simulink model "controller_dev_sg_HIL_noTP"  (R2018b)
settings: configuration reference "Physics" (kept outside this file)
model workspace (MAT data in the model file):
  m = 1000
values from neighbouring files (symbols this model uses):
  bool_activate_Vehicles : value not decoded    [controller_dev_sg.sldd]
  ModObj_ObjList_SendPort = 11004.0    [UDPPortConfig.sldd]
  ModSens_GpsSenDat_SendPort = 3002.0    [UDPPortConfig.sldd]
  sensors_freq_camera = 37.0    [controller_dev_sg.sldd]
  sensors_freq_gps = 20.0    [controller_dev_sg.sldd]
  sensors_freq_imu = 100.0    [controller_dev_sg.sldd]
  sensors_freq_lidar = 12.0    [controller_dev_sg.sldd]
  sensors_freq_radar = 20.0    [controller_dev_sg.sldd]
undefined symbols (not defined in the file or in its folder): activate_VariableFriction, C, tpa_map_Reference, tSPhysics, x0_vehiclepos_start_veh1, x0_vehiclepos_start_veh10, x0_vehiclepos_start_veh2, x0_vehiclepos_start_veh3, x0_vehiclepos_start_veh4, x0_vehiclepos_start_veh5, x0_vehiclepos_start_veh6, x0_vehiclepos_start_veh7, x0_vehiclepos_start_veh8, x0_vehiclepos_start_veh9
libraries: xpcutilitieslib x273, xpcrtudplib x215, aerolibconvert2 x48, simulink x30, etargetslib x26, speedgoatlib_IO612 x7, canmsglib x6, slrtlib x4
(part 15 of 16)

== matlab function controller_dev_sg_HIL_noTP/UDP to Sensors (GNSS, IMU)/INSPVA/grid conv angle ==
  data: lat input; gamma output; lon input
function gamma = fcn(lat, lon)

gamma = grid_conv_angle(lat, lon);

== matlab function controller_dev_sg_HIL_noTP/UDP to Sensors (GNSS, IMU)1/INSPVA/CRC32 ==
  data: data input; crc output
function crc = fcn(data)

crc = crc32(data);

== matlab function controller_dev_sg_HIL_noTP/UDP to Sensors (GNSS, IMU)/INSPVA/normalizeAngle360 ==
  data: u input; y output
function y = fcn(u)

y = normalizeAngle360(u);

== matlab function controller_dev_sg_HIL_noTP/UDP to Sensors (GNSS, IMU)1/INSPVA/Header ==
  data: id input; first output; length input; time input; leapseconds input; second output; third output; hlength output; id output; type output; port output; mlength output; seq output; idletime output; timestatus output; week output; ms output; recstatus output; reserved output; version output
function [first, second, third, hlength, id, type, port, mlength, seq, idletime, timestatus, week, ms, recstatus, reserved, version] = fcn(id, length, time, leapseconds)

[first, second, third, hlength, id, type, port, mlength, seq, idletime, timestatus, week, ms, recstatus, reserved, version] = novatel_header(id, length, time, leapseconds);

== matlab function controller_dev_sg_HIL_noTP/UDP to Sensors (GNSS, IMU)1/INSPVA/grid conv angle ==
  data: lat input; gamma output; lon input
function gamma = fcn(lat, lon)

gamma = grid_conv_angle(lat, lon);

== matlab function controller_dev_sg_HIL_noTP/UDP to Sensors (GNSS, IMU)1/INSPVA/normalizeAngle360 ==
  data: u input; y output
function y = fcn(u)

y = normalizeAngle360(u);

== matlab function controller_dev_sg_HIL_noTP/UDP to Sensors (GNSS, IMU)1/INSPVA/tcs2llhT ==
  data: x input; lat output; y input; z input; origin input; lon output; hgt output
function [lat, lon, hgt]= fcn(x, y, z, origin)

llh =tcs2llhT([x; y; z], origin);
lat = llh(1,:);
lon = llh(2,:);
hgt = llh(3,:);
end

== matlab function controller_dev_sg_HIL_noTP/UDP to Sensors (GNSS, IMU)2/INSPVA/CRC32 ==
  data: data input; crc output
function crc = fcn(data)

crc = crc32(data);

== matlab function controller_dev_sg_HIL_noTP/UDP to Sensors (GNSS, IMU)2/INSPVA/Header ==
  data: id input; first output; length input; time input; leapseconds input; second output; third output; hlength output; id output; type output; port output; mlength output; seq output; idletime output; timestatus output; week output; ms output; recstatus output; reserved output; version output
function [first, second, third, hlength, id, type, port, mlength, seq, idletime, timestatus, week, ms, recstatus, reserved, version] = fcn(id, length, time, leapseconds)

[first, second, third, hlength, id, type, port, mlength, seq, idletime, timestatus, week, ms, recstatus, reserved, version] = novatel_header(id, length, time, leapseconds);

== matlab function controller_dev_sg_HIL_noTP/UDP to Sensors (GNSS, IMU)2/INSPVA/grid conv angle ==
  data: lat input; gamma output; lon input
function gamma = fcn(lat, lon)

gamma = grid_conv_angle(lat, lon);

== matlab function controller_dev_sg_HIL_noTP/UDP to Sensors (GNSS, IMU)2/INSPVA/normalizeAngle360 ==
  data: u input; y output
function y = fcn(u)

y = normalizeAngle360(u);

== matlab function controller_dev_sg_HIL_noTP/UDP to Sensors (GNSS, IMU)2/INSPVA/tcs2llhT ==
  data: x input; lat output; y input; z input; origin input; lon output; hgt output
function [lat, lon, hgt]= fcn(x, y, z, origin)

llh =tcs2llhT([x; y; z], origin);
lat = llh(1,:);
lon = llh(2,:);
hgt = llh(3,:);
end

== matlab function controller_dev_sg_HIL_noTP/UDP to Sensors (GNSS, IMU)3/INSPVA/CRC32 ==
  data: data input; crc output
function crc = fcn(data)

crc = crc32(data);

== matlab function controller_dev_sg_HIL_noTP/UDP to Sensors (GNSS, IMU)3/INSPVA/Header ==
  data: id input; first output; length input; time input; leapseconds input; second output; third output; hlength output; id output; type output; port output; mlength output; seq output; idletime output; timestatus output; week output; ms output; recstatus output; reserved output; version output
function [first, second, third, hlength, id, type, port, mlength, seq, idletime, timestatus, week, ms, recstatus, reserved, version] = fcn(id, length, time, leapseconds)

[first, second, third, hlength, id, type, port, mlength, seq, idletime, timestatus, week, ms, recstatus, reserved, version] = novatel_header(id, length, time, leapseconds);

== matlab function controller_dev_sg_HIL_noTP/UDP to Sensors (GNSS, IMU)3/INSPVA/grid conv angle ==
  data: lat input; gamma output; lon input
function gamma = fcn(lat, lon)

gamma = grid_conv_angle(lat, lon);

== matlab function controller_dev_sg_HIL_noTP/UDP to Sensors (GNSS, IMU)3/INSPVA/normalizeAngle360 ==
  data: u input; y output
function y = fcn(u)

y = normalizeAngle360(u);

== matlab function controller_dev_sg_HIL_noTP/UDP to Sensors (GNSS, IMU)3/INSPVA/tcs2llhT ==
  data: x input; lat output; y input; z input; origin input; lon output; hgt output
function [lat, lon, hgt]= fcn(x, y, z, origin)

llh =tcs2llhT([x; y; z], origin);
lat = llh(1,:);
lon = llh(2,:);
hgt = llh(3,:);
end

== matlab function controller_dev_sg_HIL_noTP/UDP to Sensors (GNSS, IMU)4/INSPVA/CRC32 ==
  data: data input; crc output
function crc = fcn(data)

crc = crc32(data);

== matlab function controller_dev_sg_HIL_noTP/UDP to Sensors (GNSS, IMU)4/INSPVA/Header ==
  data: id input; first output; length input; time input; leapseconds input; second output; third output; hlength output; id output; type output; port output; mlength output; seq output; idletime output; timestatus output; week output; ms output; recstatus output; reserved output; version output
function [first, second, third, hlength, id, type, port, mlength, seq, idletime, timestatus, week, ms, recstatus, reserved, version] = fcn(id, length, time, leapseconds)

[first, second, third, hlength, id, type, port, mlength, seq, idletime, timestatus, week, ms, recstatus, reserved, version] = novatel_header(id, length, time, leapseconds);

== matlab function controller_dev_sg_HIL_noTP/UDP to Sensors (GNSS, IMU)4/INSPVA/grid conv angle ==
  data: lat input; gamma output; lon input
function gamma = fcn(lat, lon)

gamma = grid_conv_angle(lat, lon);

== matlab function controller_dev_sg_HIL_noTP/UDP to Sensors (GNSS, IMU)4/INSPVA/normalizeAngle360 ==
  data: u input; y output
function y = fcn(u)

y = normalizeAngle360(u);

== matlab function controller_dev_sg_HIL_noTP/UDP to Sensors (GNSS, IMU)4/INSPVA/tcs2llhT ==
  data: x input; lat output; y input; z input; origin input; lon output; hgt output
function [lat, lon, hgt]= fcn(x, y, z, origin)

llh =tcs2llhT([x; y; z], origin);
lat = llh(1,:);
lon = llh(2,:);
hgt = llh(3,:);
end

== matlab function controller_dev_sg_HIL_noTP/UDP to Sensors (GNSS, IMU)5/INSPVA/CRC32 ==
  data: data input; crc output
function crc = fcn(data)

crc = crc32(data);

== matlab function controller_dev_sg_HIL_noTP/UDP to Sensors (GNSS, IMU)5/INSPVA/Header ==
  data: id input; first output; length input; time input; leapseconds input; second output; third output; hlength output; id output; type output; port output; mlength output; seq output; idletime output; timestatus output; week output; ms output; recstatus output; reserved output; version output
function [first, second, third, hlength, id, type, port, mlength, seq, idletime, timestatus, week, ms, recstatus, reserved, version] = fcn(id, length, time, leapseconds)

[first, second, third, hlength, id, type, port, mlength, seq, idletime, timestatus, week, ms, recstatus, reserved, version] = novatel_header(id, length, time, leapseconds);

== matlab function controller_dev_sg_HIL_noTP/UDP to Sensors (GNSS, IMU)5/INSPVA/grid conv angle ==
  data: lat input; gamma output; lon input
function gamma = fcn(lat, lon)

gamma = grid_conv_angle(lat, lon);

== matlab function controller_dev_sg_HIL_noTP/UDP to Sensors (GNSS, IMU)5/INSPVA/normalizeAngle360 ==
  data: u input; y output
function y = fcn(u)

y = normalizeAngle360(u);

== matlab function controller_dev_sg_HIL_noTP/UDP to Sensors (GNSS, IMU)5/INSPVA/tcs2llhT ==
  data: x input; lat output; y input; z input; origin input; lon output; hgt output
function [lat, lon, hgt]= fcn(x, y, z, origin)

llh =tcs2llhT([x; y; z], origin);
lat = llh(1,:);
lon = llh(2,:);
hgt = llh(3,:);
end

== matlab function controller_dev_sg_HIL_noTP/UDP to Sensors (GNSS, IMU)6/INSPVA/CRC32 ==
  data: data input; crc output
function crc = fcn(data)

crc = crc32(data);

== matlab function controller_dev_sg_HIL_noTP/UDP to Sensors (GNSS, IMU)6/INSPVA/Header ==
  data: id input; first output; length input; time input; leapseconds input; second output; third output; hlength output; id output; type output; port output; mlength output; seq output; idletime output; timestatus output; week output; ms output; recstatus output; reserved output; version output
function [first, second, third, hlength, id, type, port, mlength, seq, idletime, timestatus, week, ms, recstatus, reserved, version] = fcn(id, length, time, leapseconds)

[first, second, third, hlength, id, type, port, mlength, seq, idletime, timestatus, week, ms, recstatus, reserved, version] = novatel_header(id, length, time, leapseconds);

== matlab function controller_dev_sg_HIL_noTP/UDP to Sensors (GNSS, IMU)6/INSPVA/grid conv angle ==
  data: lat input; gamma output; lon input
function gamma = fcn(lat, lon)

gamma = grid_conv_angle(lat, lon);

== matlab function controller_dev_sg_HIL_noTP/UDP to Sensors (GNSS, IMU)6/INSPVA/normalizeAngle360 ==
  data: u input; y output
function y = fcn(u)

y = normalizeAngle360(u);

== matlab function controller_dev_sg_HIL_noTP/UDP to Sensors (GNSS, IMU)6/INSPVA/tcs2llhT ==
  data: x input; lat output; y input; z input; origin input; lon output; hgt output
function [lat, lon, hgt]= fcn(x, y, z, origin)

llh =tcs2llhT([x; y; z], origin);
lat = llh(1,:);
lon = llh(2,:);
hgt = llh(3,:);
end

== matlab function controller_dev_sg_HIL_noTP/UDP to Sensors (GNSS, IMU)7/INSPVA/CRC32 ==
  data: data input; crc output
function crc = fcn(data)

crc = crc32(data);

== matlab function controller_dev_sg_HIL_noTP/UDP to Sensors (GNSS, IMU)7/INSPVA/Header ==
  data: id input; first output; length input; time input; leapseconds input; second output; third output; hlength output; id output; type output; port output; mlength output; seq output; idletime output; timestatus output; week output; ms output; recstatus output; reserved output; version output
function [first, second, third, hlength, id, type, port, mlength, seq, idletime, timestatus, week, ms, recstatus, reserved, version] = fcn(id, length, time, leapseconds)

[first, second, third, hlength, id, type, port, mlength, seq, idletime, timestatus, week, ms, recstatus, reserved, version] = novatel_header(id, length, time, leapseconds);

== matlab function controller_dev_sg_HIL_noTP/UDP to Sensors (GNSS, IMU)7/INSPVA/grid conv angle ==
  data: lat input; gamma output; lon input
function gamma = fcn(lat, lon)

gamma = grid_conv_angle(lat, lon);

== matlab function controller_dev_sg_HIL_noTP/UDP to Sensors (GNSS, IMU)7/INSPVA/normalizeAngle360 ==
  data: u input; y output
function y = fcn(u)

y = normalizeAngle360(u);

== matlab function controller_dev_sg_HIL_noTP/UDP to Sensors (GNSS, IMU)7/INSPVA/tcs2llhT ==
  data: x input; lat output; y input; z input; origin input; lon output; hgt output
function [lat, lon, hgt]= fcn(x, y, z, origin)

llh =tcs2llhT([x; y; z], origin);
lat = llh(1,:);
lon = llh(2,:);
hgt = llh(3,:);
end

== matlab function controller_dev_sg_HIL_noTP/UDP to Sensors (GNSS, IMU)/RAWIMU/CRC32 ==
  data: data input; crc output
function crc = fcn(data)

crc = crc32(data);

== matlab function controller_dev_sg_HIL_noTP/UDP to Sensors (GNSS, IMU)1/RAWIMU/CRC32 ==
  data: data input; crc output
function crc = fcn(data)

crc = crc32(data);

== matlab function controller_dev_sg_HIL_noTP/UDP to Sensors (GNSS, IMU)2/RAWIMU/CRC32 ==
  data: data input; crc output
function crc = fcn(data)

crc = crc32(data);

== matlab function controller_dev_sg_HIL_noTP/UDP to Sensors (GNSS, IMU)3/RAWIMU/CRC32 ==
  data: data input; crc output
function crc = fcn(data)

crc = crc32(data);

== matlab function controller_dev_sg_HIL_noTP/UDP to Sensors (GNSS, IMU)4/RAWIMU/CRC32 ==
  data: data input; crc output
function crc = fcn(data)

crc = crc32(data);

== matlab function controller_dev_sg_HIL_noTP/UDP to Sensors (GNSS, IMU)5/RAWIMU/CRC32 ==
  data: data input; crc output
function crc = fcn(data)

crc = crc32(data);

== matlab function controller_dev_sg_HIL_noTP/UDP to Sensors (GNSS, IMU)6/RAWIMU/CRC32 ==
  data: data input; crc output
function crc = fcn(data)

crc = crc32(data);

== matlab function controller_dev_sg_HIL_noTP/UDP to Sensors (GNSS, IMU)7/RAWIMU/CRC32 ==
  data: data input; crc output
function crc = fcn(data)

crc = crc32(data);

== matlab function controller_dev_sg_HIL_noTP/UDP to Sensors (GNSS, IMU)/BESTPOS/CRC1 ==
  data: data input; crc output
function crc = fcn(data)

crc = crc32(data);

== matlab function controller_dev_sg_HIL_noTP/UDP to Sensors (GNSS, IMU)/BESTPOS/Header1 ==
  data: id input; first output; length input; time input; leapseconds input; second output; third output; hlength output; id output; type output; port output; mlength output; seq output; idletime output; timestatus output; week output; ms output; recstatus output; reserved output; version output
function [first, second, third, hlength, id, type, port, mlength, seq, idletime, timestatus, week, ms, recstatus, reserved, version] = fcn(id, length, time, leapseconds)

[first, second, third, hlength, id, type, port, mlength, seq, idletime, timestatus, week, ms, recstatus, reserved, version] = novatel_header(id, length, time, leapseconds);

== matlab function controller_dev_sg_HIL_noTP/UDP to Sensors (GNSS, IMU)/BESTPOS/tcs2llhT1 ==
  data: x input; lat output; y input; z input; origin input; lon output; hgt output
function [lat, lon, hgt]= fcn(x, y, z, origin)

llh =tcs2llhT([x; y; z], origin);
lat = llh(1,:);
lon = llh(2,:);
hgt = llh(3,:);
end

== matlab function controller_dev_sg_HIL_noTP/UDP to Sensors (GNSS, IMU)1/BESTPOS/Header1 ==
  data: id input; first output; length input; time input; leapseconds input; second output; third output; hlength output; id output; type output; port output; mlength output; seq output; idletime output; timestatus output; week output; ms output; recstatus output; reserved output; version output
function [first, second, third, hlength, id, type, port, mlength, seq, idletime, timestatus, week, ms, recstatus, reserved, version] = fcn(id, length, time, leapseconds)

[first, second, third, hlength, id, type, port, mlength, seq, idletime, timestatus, week, ms, recstatus, reserved, version] = novatel_header(id, length, time, leapseconds);

== matlab function controller_dev_sg_HIL_noTP/UDP to Sensors (GNSS, IMU)1/BESTPOS/tcs2llhT ==
  data: x input; lat output; y input; z input; origin input; lon output; hgt output
function [lat, lon, hgt]= fcn(x, y, z, origin)

llh =tcs2llhT([x; y; z], origin);
lat = llh(1,:);
lon = llh(2,:);
hgt = llh(3,:);
end

== matlab function controller_dev_sg_HIL_noTP/UDP to Sensors (GNSS, IMU)1/BESTPOS/tcs2llhT1 ==
  data: x input; lat output; y input; z input; origin input; lon output; hgt output
function [lat, lon, hgt]= fcn(x, y, z, origin)

llh =tcs2llhT([x; y; z], origin);
lat = llh(1,:);
lon = llh(2,:);
hgt = llh(3,:);
end

== matlab function controller_dev_sg_HIL_noTP/UDP to Sensors (GNSS, IMU)2/BESTPOS/Header1 ==
  data: id input; first output; length input; time input; leapseconds input; second output; third output; hlength output; id output; type output; port output; mlength output; seq output; idletime output; timestatus output; week output; ms output; recstatus output; reserved output; version output
function [first, second, third, hlength, id, type, port, mlength, seq, idletime, timestatus, week, ms, recstatus, reserved, version] = fcn(id, length, time, leapseconds)

[first, second, third, hlength, id, type, port, mlength, seq, idletime, timestatus, week, ms, recstatus, reserved, version] = novatel_header(id, length, time, leapseconds);

== matlab function controller_dev_sg_HIL_noTP/UDP to Sensors (GNSS, IMU)2/BESTPOS/tcs2llhT ==
  data: x input; lat output; y input; z input; origin input; lon output; hgt output
function [lat, lon, hgt]= fcn(x, y, z, origin)

llh =tcs2llhT([x; y; z], origin);
lat = llh(1,:);
lon = llh(2,:);
hgt = llh(3,:);
end

== matlab function controller_dev_sg_HIL_noTP/UDP to Sensors (GNSS, IMU)2/BESTPOS/tcs2llhT1 ==
  data: x input; lat output; y input; z input; origin input; lon output; hgt output
function [lat, lon, hgt]= fcn(x, y, z, origin)

llh =tcs2llhT([x; y; z], origin);
lat = llh(1,:);
lon = llh(2,:);
hgt = llh(3,:);
end

== matlab function controller_dev_sg_HIL_noTP/UDP to Sensors (GNSS, IMU)3/BESTPOS/Header1 ==
  data: id input; first output; length input; time input; leapseconds input; second output; third output; hlength output; id output; type output; port output; mlength output; seq output; idletime output; timestatus output; week output; ms output; recstatus output; reserved output; version output
function [first, second, third, hlength, id, type, port, mlength, seq, idletime, timestatus, week, ms, recstatus, reserved, version] = fcn(id, length, time, leapseconds)

[first, second, third, hlength, id, type, port, mlength, seq, idletime, timestatus, week, ms, recstatus, reserved, version] = novatel_header(id, length, time, leapseconds);

== matlab function controller_dev_sg_HIL_noTP/UDP to Sensors (GNSS, IMU)3/BESTPOS/tcs2llhT ==
  data: x input; lat output; y input; z input; origin input; lon output; hgt output
function [lat, lon, hgt]= fcn(x, y, z, origin)

llh =tcs2llhT([x; y; z], origin);
lat = llh(1,:);
lon = llh(2,:);
hgt = llh(3,:);
end

== matlab function controller_dev_sg_HIL_noTP/UDP to Sensors (GNSS, IMU)3/BESTPOS/tcs2llhT1 ==
  data: x input; lat output; y input; z input; origin input; lon output; hgt output
function [lat, lon, hgt]= fcn(x, y, z, origin)

llh =tcs2llhT([x; y; z], origin);
lat = llh(1,:);
lon = llh(2,:);
hgt = llh(3,:);
end

== matlab function controller_dev_sg_HIL_noTP/UDP to Sensors (GNSS, IMU)4/BESTPOS/Header1 ==
  data: id input; first output; length input; time input; leapseconds input; second output; third output; hlength output; id output; type output; port output; mlength output; seq output; idletime output; timestatus output; week output; ms output; recstatus output; reserved output; version output
function [first, second, third, hlength, id, type, port, mlength, seq, idletime, timestatus, week, ms, recstatus, reserved, version] = fcn(id, length, time, leapseconds)

[first, second, third, hlength, id, type, port, mlength, seq, idletime, timestatus, week, ms, recstatus, reserved, version] = novatel_header(id, length, time, leapseconds);

== matlab function controller_dev_sg_HIL_noTP/UDP to Sensors (GNSS, IMU)4/BESTPOS/tcs2llhT ==
  data: x input; lat output; y input; z input; origin input; lon output; hgt output
function [lat, lon, hgt]= fcn(x, y, z, origin)

llh =tcs2llhT([x; y; z], origin);
lat = llh(1,:);
lon = llh(2,:);
hgt = llh(3,:);
end

== matlab function controller_dev_sg_HIL_noTP/UDP to Sensors (GNSS, IMU)4/BESTPOS/tcs2llhT1 ==
  data: x input; lat output; y input; z input; origin input; lon output; hgt output
function [lat, lon, hgt]= fcn(x, y, z, origin)

llh =tcs2llhT([x; y; z], origin);
lat = llh(1,:);
lon = llh(2,:);
hgt = llh(3,:);
end

== matlab function controller_dev_sg_HIL_noTP/UDP to Sensors (GNSS, IMU)5/BESTPOS/Header1 ==
  data: id input; first output; length input; time input; leapseconds input; second output; third output; hlength output; id output; type output; port output; mlength output; seq output; idletime output; timestatus output; week output; ms output; recstatus output; reserved output; version output
function [first, second, third, hlength, id, type, port, mlength, seq, idletime, timestatus, week, ms, recstatus, reserved, version] = fcn(id, length, time, leapseconds)

[first, second, third, hlength, id, type, port, mlength, seq, idletime, timestatus, week, ms, recstatus, reserved, version] = novatel_header(id, length, time, leapseconds);

== matlab function controller_dev_sg_HIL_noTP/UDP to Sensors (GNSS, IMU)5/BESTPOS/tcs2llhT ==
  data: x input; lat output; y input; z input; origin input; lon output; hgt output
function [lat, lon, hgt]= fcn(x, y, z, origin)

llh =tcs2llhT([x; y; z], origin);
lat = llh(1,:);
lon = llh(2,:);
hgt = llh(3,:);
end

== matlab function controller_dev_sg_HIL_noTP/UDP to Sensors (GNSS, IMU)5/BESTPOS/tcs2llhT1 ==
  data: x input; lat output; y input; z input; origin input; lon output; hgt output
function [lat, lon, hgt]= fcn(x, y, z, origin)

llh =tcs2llhT([x; y; z], origin);
lat = llh(1,:);
lon = llh(2,:);
hgt = llh(3,:);
end

== matlab function controller_dev_sg_HIL_noTP/UDP to Sensors (GNSS, IMU)6/BESTPOS/Header1 ==
  data: id input; first output; length input; time input; leapseconds input; second output; third output; hlength output; id output; type output; port output; mlength output; seq output; idletime output; timestatus output; week output; ms output; recstatus output; reserved output; version output
function [first, second, third, hlength, id, type, port, mlength, seq, idletime, timestatus, week, ms, recstatus, reserved, version] = fcn(id, length, time, leapseconds)

[first, second, third, hlength, id, type, port, mlength, seq, idletime, timestatus, week, ms, recstatus, reserved, version] = novatel_header(id, length, time, leapseconds);

== matlab function controller_dev_sg_HIL_noTP/UDP to Sensors (GNSS, IMU)6/BESTPOS/tcs2llhT ==
  data: x input; lat output; y input; z input; origin input; lon output; hgt output
function [lat, lon, hgt]= fcn(x, y, z, origin)

llh =tcs2llhT([x; y; z], origin);
lat = llh(1,:);
lon = llh(2,:);
hgt = llh(3,:);
end

== matlab function controller_dev_sg_HIL_noTP/UDP to Sensors (GNSS, IMU)6/BESTPOS/tcs2llhT1 ==
  data: x input; lat output; y input; z input; origin input; lon output; hgt output
function [lat, lon, hgt]= fcn(x, y, z, origin)

llh =tcs2llhT([x; y; z], origin);
lat = llh(1,:);
lon = llh(2,:);
hgt = llh(3,:);
end

== matlab function controller_dev_sg_HIL_noTP/UDP to Sensors (GNSS, IMU)7/BESTPOS/Header1 ==
  data: id input; first output; length input; time input; leapseconds input; second output; third output; hlength output; id output; type output; port output; mlength output; seq output; idletime output; timestatus output; week output; ms output; recstatus output; reserved output; version output
function [first, second, third, hlength, id, type, port, mlength, seq, idletime, timestatus, week, ms, recstatus, reserved, version] = fcn(id, length, time, leapseconds)

[first, second, third, hlength, id, type, port, mlength, seq, idletime, timestatus, week, ms, recstatus, reserved, version] = novatel_header(id, length, time, leapseconds);

== matlab function controller_dev_sg_HIL_noTP/UDP to Sensors (GNSS, IMU)7/BESTPOS/tcs2llhT ==
  data: x input; lat output; y input; z input; origin input; lon output; hgt output
function [lat, lon, hgt]= fcn(x, y, z, origin)

llh =tcs2llhT([x; y; z], origin);
lat = llh(1,:);
lon = llh(2,:);
hgt = llh(3,:);
end

== matlab function controller_dev_sg_HIL_noTP/UDP to Sensors (GNSS, IMU)7/BESTPOS/tcs2llhT1 ==
  data: x input; lat output; y input; z input; origin input; lon output; hgt output
function [lat, lon, hgt]= fcn(x, y, z, origin)

llh =tcs2llhT([x; y; z], origin);
lat = llh(1,:);
lon = llh(2,:);
hgt = llh(3,:);
end

== matlab function controller_dev_sg_HIL_noTP/UDP to Sensors (GNSS, IMU)/DUALANTENNAHEADING/CRC32 ==
  data: data input; crc output
function crc = fcn(data)

crc = crc32(data);

== matlab function controller_dev_sg_HIL_noTP/UDP to Sensors (GNSS, IMU)/DUALANTENNAHEADING/Header ==
  data: id input; first output; length input; time input; leapseconds input; second output; third output; hlength output; id output; type output; port output; mlength output; seq output; idletime output; timestatus output; week output; ms output; recstatus output; reserved output; version output
function [first, second, third, hlength, id, type, port, mlength, seq, idletime, timestatus, week, ms, recstatus, reserved, version] = fcn(id, length, time, leapseconds)

[first, second, third, hlength, id, type, port, mlength, seq, idletime, timestatus, week, ms, recstatus, reserved, version] = novatel_header(id, length, time, leapseconds);

== matlab function controller_dev_sg_HIL_noTP/UDP to Sensors (GNSS, IMU)/DUALANTENNAHEADING/grid conv angle ==
  data: lat input; gamma output; lon input
function gamma = fcn(lat, lon)

gamma = grid_conv_angle(lat, lon);

== matlab function controller_dev_sg_HIL_noTP/UDP to Sensors (GNSS, IMU)/DUALANTENNAHEADING/normalizeAngle360 ==
  data: u input; y output
function y = fcn(u)

y = normalizeAngle360(u);

== matlab function controller_dev_sg_HIL_noTP/UDP to Sensors (GNSS, IMU)/DUALANTENNAHEADING/tcs2llhT ==
  data: x input; lat output; y input; z input; origin input; lon output; hgt output
function [lat, lon, hgt]= fcn(x, y, z, origin)

llh =tcs2llhT([x; y; z], origin);
lat = llh(1,:);
lon = llh(2,:);
hgt = llh(3,:);
end

== matlab function controller_dev_sg_HIL_noTP/UDP to Sensors (GNSS, IMU)1/DUALANTENNAHEADING/CRC32 ==
  data: data input; crc output
function crc = fcn(data)

crc = crc32(data);

== matlab function controller_dev_sg_HIL_noTP/UDP to Sensors (GNSS, IMU)1/DUALANTENNAHEADING/Header ==
  data: id input; first output; length input; time input; leapseconds input; second output; third output; hlength output; id output; type output; port output; mlength output; seq output; idletime output; timestatus output; week output; ms output; recstatus output; reserved output; version output
function [first, second, third, hlength, id, type, port, mlength, seq, idletime, timestatus, week, ms, recstatus, reserved, version] = fcn(id, length, time, leapseconds)

[first, second, third, hlength, id, type, port, mlength, seq, idletime, timestatus, week, ms, recstatus, reserved, version] = novatel_header(id, length, time, leapseconds);

== matlab function controller_dev_sg_HIL_noTP/UDP to Sensors (GNSS, IMU)1/DUALANTENNAHEADING/grid conv angle ==
  data: lat input; gamma output; lon input
function gamma = fcn(lat, lon)

gamma = grid_conv_angle(lat, lon);

== matlab function controller_dev_sg_HIL_noTP/UDP to Sensors (GNSS, IMU)1/DUALANTENNAHEADING/normalizeAngle360 ==
  data: u input; y output
function y = fcn(u)

y = normalizeAngle360(u);

== matlab function controller_dev_sg_HIL_noTP/UDP to Sensors (GNSS, IMU)1/DUALANTENNAHEADING/tcs2llhT ==
  data: x input; lat output; y input; z input; origin input; lon output; hgt output
function [lat, lon, hgt]= fcn(x, y, z, origin)

llh =tcs2llhT([x; y; z], origin);
lat = llh(1,:);
lon = llh(2,:);
hgt = llh(3,:);
end

== matlab function controller_dev_sg_HIL_noTP/UDP to Sensors (GNSS, IMU)2/DUALANTENNAHEADING/CRC32 ==
  data: data input; crc output
function crc = fcn(data)

crc = crc32(data);

== matlab function controller_dev_sg_HIL_noTP/UDP to Sensors (GNSS, IMU)2/DUALANTENNAHEADING/Header ==
  data: id input; first output; length input; time input; leapseconds input; second output; third output; hlength output; id output; type output; port output; mlength output; seq output; idletime output; timestatus output; week output; ms output; recstatus output; reserved output; version output
function [first, second, third, hlength, id, type, port, mlength, seq, idletime, timestatus, week, ms, recstatus, reserved, version] = fcn(id, length, time, leapseconds)

[first, second, third, hlength, id, type, port, mlength, seq, idletime, timestatus, week, ms, recstatus, reserved, version] = novatel_header(id, length, time, leapseconds);

== matlab function controller_dev_sg_HIL_noTP/UDP to Sensors (GNSS, IMU)2/DUALANTENNAHEADING/grid conv angle ==
  data: lat input; gamma output; lon input
function gamma = fcn(lat, lon)

gamma = grid_conv_angle(lat, lon);

== matlab function controller_dev_sg_HIL_noTP/UDP to Sensors (GNSS, IMU)2/DUALANTENNAHEADING/normalizeAngle360 ==
  data: u input; y output
function y = fcn(u)

y = normalizeAngle360(u);

== matlab function controller_dev_sg_HIL_noTP/UDP to Sensors (GNSS, IMU)2/DUALANTENNAHEADING/tcs2llhT ==
  data: x input; lat output; y input; z input; origin input; lon output; hgt output
function [lat, lon, hgt]= fcn(x, y, z, origin)

llh =tcs2llhT([x; y; z], origin);
lat = llh(1,:);
lon = llh(2,:);
hgt = llh(3,:);
end

== matlab function controller_dev_sg_HIL_noTP/UDP to Sensors (GNSS, IMU)3/DUALANTENNAHEADING/CRC32 ==
  data: data input; crc output
function crc = fcn(data)

crc = crc32(data);

== matlab function controller_dev_sg_HIL_noTP/UDP to Sensors (GNSS, IMU)3/DUALANTENNAHEADING/Header ==
  data: id input; first output; length input; time input; leapseconds input; second output; third output; hlength output; id output; type output; port output; mlength output; seq output; idletime output; timestatus output; week output; ms output; recstatus output; reserved output; version output
function [first, second, third, hlength, id, type, port, mlength, seq, idletime, timestatus, week, ms, recstatus, reserved, version] = fcn(id, length, time, leapseconds)

[first, second, third, hlength, id, type, port, mlength, seq, idletime, timestatus, week, ms, recstatus, reserved, version] = novatel_header(id, length, time, leapseconds);

== matlab function controller_dev_sg_HIL_noTP/UDP to Sensors (GNSS, IMU)3/DUALANTENNAHEADING/grid conv angle ==
  data: lat input; gamma output; lon input
function gamma = fcn(lat, lon)

gamma = grid_conv_angle(lat, lon);

== matlab function controller_dev_sg_HIL_noTP/UDP to Sensors (GNSS, IMU)3/DUALANTENNAHEADING/normalizeAngle360 ==
  data: u input; y output
function y = fcn(u)

y = normalizeAngle360(u);

== matlab function controller_dev_sg_HIL_noTP/UDP to Sensors (GNSS, IMU)3/DUALANTENNAHEADING/tcs2llhT ==
  data: x input; lat output; y input; z input; origin input; lon output; hgt output
function [lat, lon, hgt]= fcn(x, y, z, origin)

llh =tcs2llhT([x; y; z], origin);
lat = llh(1,:);
lon = llh(2,:);
hgt = llh(3,:);
end

== matlab function controller_dev_sg_HIL_noTP/UDP to Sensors (GNSS, IMU)4/DUALANTENNAHEADING/CRC32 ==
  data: data input; crc output
function crc = fcn(data)

crc = crc32(data);

== matlab function controller_dev_sg_HIL_noTP/UDP to Sensors (GNSS, IMU)4/DUALANTENNAHEADING/Header ==
  data: id input; first output; length input; time input; leapseconds input; second output; third output; hlength output; id output; type output; port output; mlength output; seq output; idletime output; timestatus output; week output; ms output; recstatus output; reserved output; version output
function [first, second, third, hlength, id, type, port, mlength, seq, idletime, timestatus, week, ms, recstatus, reserved, version] = fcn(id, length, time, leapseconds)

[first, second, third, hlength, id, type, port, mlength, seq, idletime, timestatus, week, ms, recstatus, reserved, version] = novatel_header(id, length, time, leapseconds);

== matlab function controller_dev_sg_HIL_noTP/UDP to Sensors (GNSS, IMU)4/DUALANTENNAHEADING/grid conv angle ==
  data: lat input; gamma output; lon input
function gamma = fcn(lat, lon)

gamma = grid_conv_angle(lat, lon);

== matlab function controller_dev_sg_HIL_noTP/UDP to Sensors (GNSS, IMU)4/DUALANTENNAHEADING/normalizeAngle360 ==
  data: u input; y output
function y = fcn(u)

y = normalizeAngle360(u);

== matlab function controller_dev_sg_HIL_noTP/UDP to Sensors (GNSS, IMU)4/DUALANTENNAHEADING/tcs2llhT ==
  data: x input; lat output; y input; z input; origin input; lon output; hgt output
function [lat, lon, hgt]= fcn(x, y, z, origin)

llh =tcs2llhT([x; y; z], origin);
lat = llh(1,:);
lon = llh(2,:);
hgt = llh(3,:);
end

== matlab function controller_dev_sg_HIL_noTP/UDP to Sensors (GNSS, IMU)5/DUALANTENNAHEADING/CRC32 ==
  data: data input; crc output
function crc = fcn(data)

crc = crc32(data);

== matlab function controller_dev_sg_HIL_noTP/UDP to Sensors (GNSS, IMU)5/DUALANTENNAHEADING/Header ==
  data: id input; first output; length input; time input; leapseconds input; second output; third output; hlength output; id output; type output; port output; mlength output; seq output; idletime output; timestatus output; week output; ms output; recstatus output; reserved output; version output
function [first, second, third, hlength, id, type, port, mlength, seq, idletime, timestatus, week, ms, recstatus, reserved, version] = fcn(id, length, time, leapseconds)

[first, second, third, hlength, id, type, port, mlength, seq, idletime, timestatus, week, ms, recstatus, reserved, version] = novatel_header(id, length, time, leapseconds);

== matlab function controller_dev_sg_HIL_noTP/UDP to Sensors (GNSS, IMU)5/DUALANTENNAHEADING/grid conv angle ==
  data: lat input; gamma output; lon input
function gamma = fcn(lat, lon)

gamma = grid_conv_angle(lat, lon);

== matlab function controller_dev_sg_HIL_noTP/UDP to Sensors (GNSS, IMU)5/DUALANTENNAHEADING/normalizeAngle360 ==
  data: u input; y output
function y = fcn(u)

y = normalizeAngle360(u);

== matlab function controller_dev_sg_HIL_noTP/UDP to Sensors (GNSS, IMU)5/DUALANTENNAHEADING/tcs2llhT ==
  data: x input; lat output; y input; z input; origin input; lon output; hgt output
function [lat, lon, hgt]= fcn(x, y, z, origin)

llh =tcs2llhT([x; y; z], origin);
lat = llh(1,:);
lon = llh(2,:);
hgt = llh(3,:);
end

== matlab function controller_dev_sg_HIL_noTP/UDP to Sensors (GNSS, IMU)6/DUALANTENNAHEADING/CRC32 ==
  data: data input; crc output
function crc = fcn(data)

crc = crc32(data);

== matlab function controller_dev_sg_HIL_noTP/UDP to Sensors (GNSS, IMU)6/DUALANTENNAHEADING/Header ==
  data: id input; first output; length input; time input; leapseconds input; second output; third output; hlength output; id output; type output; port output; mlength output; seq output; idletime output; timestatus output; week output; ms output; recstatus output; reserved output; version output
function [first, second, third, hlength, id, type, port, mlength, seq, idletime, timestatus, week, ms, recstatus, reserved, version] = fcn(id, length, time, leapseconds)

[first, second, third, hlength, id, type, port, mlength, seq, idletime, timestatus, week, ms, recstatus, reserved, version] = novatel_header(id, length, time, leapseconds);

== matlab function controller_dev_sg_HIL_noTP/UDP to Sensors (GNSS, IMU)6/DUALANTENNAHEADING/grid conv angle ==
  data: lat input; gamma output; lon input
function gamma = fcn(lat, lon)

gamma = grid_conv_angle(lat, lon);

== matlab function controller_dev_sg_HIL_noTP/UDP to Sensors (GNSS, IMU)6/DUALANTENNAHEADING/normalizeAngle360 ==
  data: u input; y output
function y = fcn(u)

y = normalizeAngle360(u);

== matlab function controller_dev_sg_HIL_noTP/UDP to Sensors (GNSS, IMU)6/DUALANTENNAHEADING/tcs2llhT ==
  data: x input; lat output; y input; z input; origin input; lon output; hgt output
function [lat, lon, hgt]= fcn(x, y, z, origin)

llh =tcs2llhT([x; y; z], origin);
lat = llh(1,:);
lon = llh(2,:);
hgt = llh(3,:);
end

== matlab function controller_dev_sg_HIL_noTP/UDP to Sensors (GNSS, IMU)7/DUALANTENNAHEADING/CRC32 ==
  data: data input; crc output
function crc = fcn(data)

crc = crc32(data);

== matlab function controller_dev_sg_HIL_noTP/UDP to Sensors (GNSS, IMU)7/DUALANTENNAHEADING/Header ==
  data: id input; first output; length input; time input; leapseconds input; second output; third output; hlength output; id output; type output; port output; mlength output; seq output; idletime output; timestatus output; week output; ms output; recstatus output; reserved output; version output
function [first, second, third, hlength, id, type, port, mlength, seq, idletime, timestatus, week, ms, recstatus, reserved, version] = fcn(id, length, time, leapseconds)

[first, second, third, hlength, id, type, port, mlength, seq, idletime, timestatus, week, ms, recstatus, reserved, version] = novatel_header(id, length, time, leapseconds);

== matlab function controller_dev_sg_HIL_noTP/UDP to Sensors (GNSS, IMU)7/DUALANTENNAHEADING/grid conv angle ==
  data: lat input; gamma output; lon input
function gamma = fcn(lat, lon)

gamma = grid_conv_angle(lat, lon);

== matlab function controller_dev_sg_HIL_noTP/UDP to Sensors (GNSS, IMU)7/DUALANTENNAHEADING/normalizeAngle360 ==
  data: u input; y output
function y = fcn(u)

y = normalizeAngle360(u);

== matlab function controller_dev_sg_HIL_noTP/UDP to Sensors (GNSS, IMU)7/DUALANTENNAHEADING/tcs2llhT ==
  data: x input; lat output; y input; z input; origin input; lon output; hgt output
function [lat, lon, hgt]= fcn(x, y, z, origin)

llh =tcs2llhT([x; y; z], origin);
lat = llh(1,:);
lon = llh(2,:);
hgt = llh(3,:);
end

== matlab function controller_dev_sg_HIL_noTP/UDP to Sensors (GNSS, IMU)/DUALANTENNAHEADING/CRC1 ==
  data: data input; crc output
function crc = fcn(data)

crc = crc32(data);

== matlab function controller_dev_sg_HIL_noTP/UDP to Sensors (GNSS, IMU)/DUALANTENNAHEADING/Header1 ==
  data: id input; first output; length input; time input; leapseconds input; second output; third output; hlength output; id output; type output; port output; mlength output; seq output; idletime output; timestatus output; week output; ms output; recstatus output; reserved output; version output
function [first, second, third, hlength, id, type, port, mlength, seq, idletime, timestatus, week, ms, recstatus, reserved, version] = fcn(id, length, time, leapseconds)

[first, second, third, hlength, id, type, port, mlength, seq, idletime, timestatus, week, ms, recstatus, reserved, version] = novatel_header(id, length, time, leapseconds);

== matlab function controller_dev_sg_HIL_noTP/UDP to Sensors (GNSS, IMU)/DUALANTENNAHEADING/grid conv angle1 ==
  data: lat input; gamma output; lon input
function gamma = fcn(lat, lon)

gamma = grid_conv_angle(lat, lon);

== matlab function controller_dev_sg_HIL_noTP/UDP to Sensors (GNSS, IMU)/DUALANTENNAHEADING/normalizeAngle1 ==
  data: u input; y output
function y = fcn(u)

y = normalizeAngle360(u);

== matlab function controller_dev_sg_HIL_noTP/UDP to Sensors (GNSS, IMU)/DUALANTENNAHEADING/tcs2llhT1 ==
  data: x input; lat output; y input; z input; origin input; lon output; hgt output
function [lat, lon, hgt]= fcn(x, y, z, origin)

llh =tcs2llhT([x; y; z], origin);
lat = llh(1,:);
lon = llh(2,:);
hgt = llh(3,:);
end

== matlab function controller_dev_sg_HIL_noTP/UDP to Sensors (GNSS, IMU)1/DUALANTENNAHEADING/CRC1 ==
  data: data input; crc output
function crc = fcn(data)

crc = crc32(data);

== matlab function controller_dev_sg_HIL_noTP/UDP to Sensors (GNSS, IMU)1/DUALANTENNAHEADING/Header1 ==
  data: id input; first output; length input; time input; leapseconds input; second output; third output; hlength output; id output; type output; port output; mlength output; seq output; idletime output; timestatus output; week output; ms output; recstatus output; reserved output; version output
function [first, second, third, hlength, id, type, port, mlength, seq, idletime, timestatus, week, ms, recstatus, reserved, version] = fcn(id, length, time, leapseconds)

[first, second, third, hlength, id, type, port, mlength, seq, idletime, timestatus, week, ms, recstatus, reserved, version] = novatel_header(id, length, time, leapseconds);

== matlab function controller_dev_sg_HIL_noTP/UDP to Sensors (GNSS, IMU)1/DUALANTENNAHEADING/grid conv angle1 ==
  data: lat input; gamma output; lon input
function gamma = fcn(lat, lon)

gamma = grid_conv_angle(lat, lon);

== matlab function controller_dev_sg_HIL_noTP/UDP to Sensors (GNSS, IMU)1/DUALANTENNAHEADING/normalizeAngle1 ==
  data: u input; y output
function y = fcn(u)

y = normalizeAngle360(u);

== matlab function controller_dev_sg_HIL_noTP/UDP to Sensors (GNSS, IMU)1/DUALANTENNAHEADING/tcs2llhT1 ==
  data: x input; lat output; y input; z input; origin input; lon output; hgt output
function [lat, lon, hgt]= fcn(x, y, z, origin)

llh =tcs2llhT([x; y; z], origin);
lat = llh(1,:);
lon = llh(2,:);
hgt = llh(3,:);
end

== matlab function controller_dev_sg_HIL_noTP/UDP to Sensors (GNSS, IMU)2/DUALANTENNAHEADING/CRC1 ==
  data: data input; crc output
function crc = fcn(data)

crc = crc32(data);

== matlab function controller_dev_sg_HIL_noTP/UDP to Sensors (GNSS, IMU)2/DUALANTENNAHEADING/Header1 ==
  data: id input; first output; length input; time input; leapseconds input; second output; third output; hlength output; id output; type output; port output; mlength output; seq output; idletime output; timestatus output; week output; ms output; recstatus output; reserved output; version output
function [first, second, third, hlength, id, type, port, mlength, seq, idletime, timestatus, week, ms, recstatus, reserved, version] = fcn(id, length, time, leapseconds)

[first, second, third, hlength, id, type, port, mlength, seq, idletime, timestatus, week, ms, recstatus, reserved, version] = novatel_header(id, length, time, leapseconds);

== matlab function controller_dev_sg_HIL_noTP/UDP to Sensors (GNSS, IMU)2/DUALANTENNAHEADING/grid conv angle1 ==
  data: lat input; gamma output; lon input
function gamma = fcn(lat, lon)

gamma = grid_conv_angle(lat, lon);

== matlab function controller_dev_sg_HIL_noTP/UDP to Sensors (GNSS, IMU)2/DUALANTENNAHEADING/normalizeAngle1 ==
  data: u input; y output
function y = fcn(u)

y = normalizeAngle360(u);

== matlab function controller_dev_sg_HIL_noTP/UDP to Sensors (GNSS, IMU)2/DUALANTENNAHEADING/tcs2llhT1 ==
  data: x input; lat output; y input; z input; origin input; lon output; hgt output
function [lat, lon, hgt]= fcn(x, y, z, origin)

llh =tcs2llhT([x; y; z], origin);
lat = llh(1,:);
lon = llh(2,:);
hgt = llh(3,:);
end

== matlab function controller_dev_sg_HIL_noTP/UDP to Sensors (GNSS, IMU)3/DUALANTENNAHEADING/CRC1 ==
  data: data input; crc output
function crc = fcn(data)

crc = crc32(data);

== matlab function controller_dev_sg_HIL_noTP/UDP to Sensors (GNSS, IMU)3/DUALANTENNAHEADING/Header1 ==
  data: id input; first output; length input; time input; leapseconds input; second output; third output; hlength output; id output; type output; port output; mlength output; seq output; idletime output; timestatus output; week output; ms output; recstatus output; reserved output; version output
function [first, second, third, hlength, id, type, port, mlength, seq, idletime, timestatus, week, ms, recstatus, reserved, version] = fcn(id, length, time, leapseconds)

[first, second, third, hlength, id, type, port, mlength, seq, idletime, timestatus, week, ms, recstatus, reserved, version] = novatel_header(id, length, time, leapseconds);

== matlab function controller_dev_sg_HIL_noTP/UDP to Sensors (GNSS, IMU)3/DUALANTENNAHEADING/grid conv angle1 ==
  data: lat input; gamma output; lon input
function gamma = fcn(lat, lon)

gamma = grid_conv_angle(lat, lon);

== matlab function controller_dev_sg_HIL_noTP/UDP to Sensors (GNSS, IMU)3/DUALANTENNAHEADING/normalizeAngle1 ==
  data: u input; y output
function y = fcn(u)

y = normalizeAngle360(u);

== matlab function controller_dev_sg_HIL_noTP/UDP to Sensors (GNSS, IMU)3/DUALANTENNAHEADING/tcs2llhT1 ==
  data: x input; lat output; y input; z input; origin input; lon output; hgt output
function [lat, lon, hgt]= fcn(x, y, z, origin)

llh =tcs2llhT([x; y; z], origin);
lat = llh(1,:);
lon = llh(2,:);
hgt = llh(3,:);
end

== matlab function controller_dev_sg_HIL_noTP/UDP to Sensors (GNSS, IMU)4/DUALANTENNAHEADING/CRC1 ==
  data: data input; crc output
function crc = fcn(data)

crc = crc32(data);

== matlab function controller_dev_sg_HIL_noTP/UDP to Sensors (GNSS, IMU)4/DUALANTENNAHEADING/Header1 ==
  data: id input; first output; length input; time input; leapseconds input; second output; third output; hlength output; id output; type output; port output; mlength output; seq output; idletime output; timestatus output; week output; ms output; recstatus output; reserved output; version output
function [first, second, third, hlength, id, type, port, mlength, seq, idletime, timestatus, week, ms, recstatus, reserved, version] = fcn(id, length, time, leapseconds)

[first, second, third, hlength, id, type, port, mlength, seq, idletime, timestatus, week, ms, recstatus, reserved, version] = novatel_header(id, length, time, leapseconds);

== matlab function controller_dev_sg_HIL_noTP/UDP to Sensors (GNSS, IMU)4/DUALANTENNAHEADING/grid conv angle1 ==
  data: lat input; gamma output; lon input
function gamma = fcn(lat, lon)

gamma = grid_conv_angle(lat, lon);

== matlab function controller_dev_sg_HIL_noTP/UDP to Sensors (GNSS, IMU)4/DUALANTENNAHEADING/normalizeAngle1 ==
  data: u input; y output
function y = fcn(u)

y = normalizeAngle360(u);

== matlab function controller_dev_sg_HIL_noTP/UDP to Sensors (GNSS, IMU)4/DUALANTENNAHEADING/tcs2llhT1 ==
  data: x input; lat output; y input; z input; origin input; lon output; hgt output
function [lat, lon, hgt]= fcn(x, y, z, origin)

llh =tcs2llhT([x; y; z], origin);
lat = llh(1,:);
lon = llh(2,:);
hgt = llh(3,:);
end

== matlab function controller_dev_sg_HIL_noTP/UDP to Sensors (GNSS, IMU)5/DUALANTENNAHEADING/CRC1 ==
  data: data input; crc output
function crc = fcn(data)

crc = crc32(data);

== matlab function controller_dev_sg_HIL_noTP/UDP to Sensors (GNSS, IMU)5/DUALANTENNAHEADING/Header1 ==
  data: id input; first output; length input; time input; leapseconds input; second output; third output; hlength output; id output; type output; port output; mlength output; seq output; idletime output; timestatus output; week output; ms output; recstatus output; reserved output; version output
function [first, second, third, hlength, id, type, port, mlength, seq, idletime, timestatus, week, ms, recstatus, reserved, version] = fcn(id, length, time, leapseconds)

[first, second, third, hlength, id, type, port, mlength, seq, idletime, timestatus, week, ms, recstatus, reserved, version] = novatel_header(id, length, time, leapseconds);

== matlab function controller_dev_sg_HIL_noTP/UDP to Sensors (GNSS, IMU)5/DUALANTENNAHEADING/grid conv angle1 ==
  data: lat input; gamma output; lon input
function gamma = fcn(lat, lon)

gamma = grid_conv_angle(lat, lon);

== matlab function controller_dev_sg_HIL_noTP/UDP to Sensors (GNSS, IMU)5/DUALANTENNAHEADING/normalizeAngle1 ==
  data: u input; y output
function y = fcn(u)

y = normalizeAngle360(u);

== matlab function controller_dev_sg_HIL_noTP/UDP to Sensors (GNSS, IMU)5/DUALANTENNAHEADING/tcs2llhT1 ==
  data: x input; lat output; y input; z input; origin input; lon output; hgt output
function [lat, lon, hgt]= fcn(x, y, z, origin)

llh =tcs2llhT([x; y; z], origin);
lat = llh(1,:);
lon = llh(2,:);
hgt = llh(3,:);
end

== matlab function controller_dev_sg_HIL_noTP/UDP to Sensors (GNSS, IMU)6/DUALANTENNAHEADING/CRC1 ==
  data: data input; crc output
function crc = fcn(data)

crc = crc32(data);

== matlab function controller_dev_sg_HIL_noTP/UDP to Sensors (GNSS, IMU)6/DUALANTENNAHEADING/Header1 ==
  data: id input; first output; length input; time input; leapseconds input; second output; third output; hlength output; id output; type output; port output; mlength output; seq output; idletime output; timestatus output; week output; ms output; recstatus output; reserved output; version output
function [first, second, third, hlength, id, type, port, mlength, seq, idletime, timestatus, week, ms, recstatus, reserved, version] = fcn(id, length, time, leapseconds)

[first, second, third, hlength, id, type, port, mlength, seq, idletime, timestatus, week, ms, recstatus, reserved, version] = novatel_header(id, length, time, leapseconds);

== matlab function controller_dev_sg_HIL_noTP/UDP to Sensors (GNSS, IMU)6/DUALANTENNAHEADING/grid conv angle1 ==
  data: lat input; gamma output; lon input
function gamma = fcn(lat, lon)

gamma = grid_conv_angle(lat, lon);

== matlab function controller_dev_sg_HIL_noTP/UDP to Sensors (GNSS, IMU)6/DUALANTENNAHEADING/normalizeAngle1 ==
  data: u input; y output
function y = fcn(u)

y = normalizeAngle360(u);

== matlab function controller_dev_sg_HIL_noTP/UDP to Sensors (GNSS, IMU)6/DUALANTENNAHEADING/tcs2llhT1 ==
  data: x input; lat output; y input; z input; origin input; lon output; hgt output
function [lat, lon, hgt]= fcn(x, y, z, origin)

llh =tcs2llhT([x; y; z], origin);
lat = llh(1,:);
lon = llh(2,:);
hgt = llh(3,:);
end
